simulink model "twoaxis_camera_gantry_start"  (R2021b)
settings: Solver=VariableStepAuto  StartTime=0.0  StopTime=inf  MaxStep=0.01  RelTol=1e-3  AbsTol=0.001  EnableMultiTasking=on
model workspace: external: MATLAB File gantryParams.m (data not in the file)
values from neighbouring files (symbols this model uses):
  endSupport = struct    [gantryParams.m]
  endSupportZ = struct    [gantryParams.m]
  leadScrew = struct    [gantryParams.m]
  leadScrewZ = struct    [gantryParams.m]
  rail = struct    [gantryParams.m]
  railZ = struct    [gantryParams.m]
  runner = struct    [gantryParams.m]
  runnerZ = struct    [gantryParams.m]
undefined symbols (not defined in the file or in its folder): DiscIntNeverNeededParam, X, Y, Z
libraries: sm_lib x81, nesl_utility x30, fl_lib x26, sm_linear_actuator_lib x14, ee_lib x4, slpidlib x2, mspsensorlib x1
(part 5 of 5)

== system twoaxis_camera_gantry_start/DC Motor z/H Bridge/Subsystem3 ==
  Constant : Constant  Value=0.5
  PS Gain : fl_lib/Physical Signals/Functions/PS Gain  gain=-1
  PS Subtract1 : fl_lib/Physical Signals/Functions/PS Subtract
  Simulink-PS Converter1 : nesl_utility/Simulink-PS Converter  PhysicalDomain=network_engine_domain  SubClassName=ps_input  LeftPortType=input  RightPortType=output  PseudoPeriodic=off  Frequencies=[]  NoiseDistribution=none  NoiseParameters=[]  Unit=1  AffineConversion=off  FilteringAndDerivatives=zero  SimscapeFilterOrder=1  InputFilterTimeConstant=.001  UdotUserProvided=0
      settings: SourceProductBaseCode=PW,SS
  Conn1 : PMIOPort  Side=Left
  Conn2 : PMIOPort  Port=2  Side=Right
  wires:
  Constant/1 -> Simulink-PS Converter1/1
  connections:
  PS Subtract1/LConn2 -- Simulink-PS Converter1/RConn1
  PS Subtract1/LConn1 -- Conn1/RConn1
  PS Gain/LConn1 -- PS Subtract1/RConn1
  PS Gain/RConn1 -- Conn2/RConn1

== matlab function twoaxis_camera_gantry_start/Controller/MATLAB Function ==
  data: position input; override output
% Z axis Vertical
% Start : 0.375
% Top: 0.545
% Min: 0.03
% Safety Lim:
% Top: 0.54
% Min: 0.04
% Middle 0.29+- 0.25

function override = fcn(position)

if position > 0.54*1.1
    override = -100;
elseif  position < 0.03
    override = 100;
else 
    override = 0;
end

== matlab function twoaxis_camera_gantry_start/Controller/MATLAB Function1 ==
  data: position input; override output
% Y axis Lateral
% Start : 0.218
% Top: 0.357
% Min: 0.02
% Safety Lim:
% Top: 0.35
% Min: 0.03
% Midle: 0.19 +- 0.16
 

function override = fcn(position)

if position > 0.35*1.05
    override = -100;
elseif  position < 0.02
    override = 100;
else 
    override = 0;
end
